simulink model "untitled"  (Simulink 8.7)
settings: Solver=VariableStepAuto  StartTime=0.0  StopTime=3  RelTol=1e-3
libraries: simulink x8
settings Model: Creator=33105  LastModifiedBy=33105
settings DataIOCC: LimitDataPoints=off  SaveFormat=Dataset
settings DebuggingCC: UnderspecifiedInitializationDetection=Simplified  MergeDetectMultiDrivingBlocksExec=error
settings HardwareCC: ProdBitPerPointer=64  ProdLargestAtomicFloat=Float  ProdIntDivRoundTo=Zero  ProdEndianess=LittleEndian  ProdWordSize=64  ProdHWDeviceType=Intel->x86-64 (Windows64)
settings ModelReferenceCC: PropagateSignalLabelsOutOfModel=on
settings ConfigComp: CovModelRefEnable=off

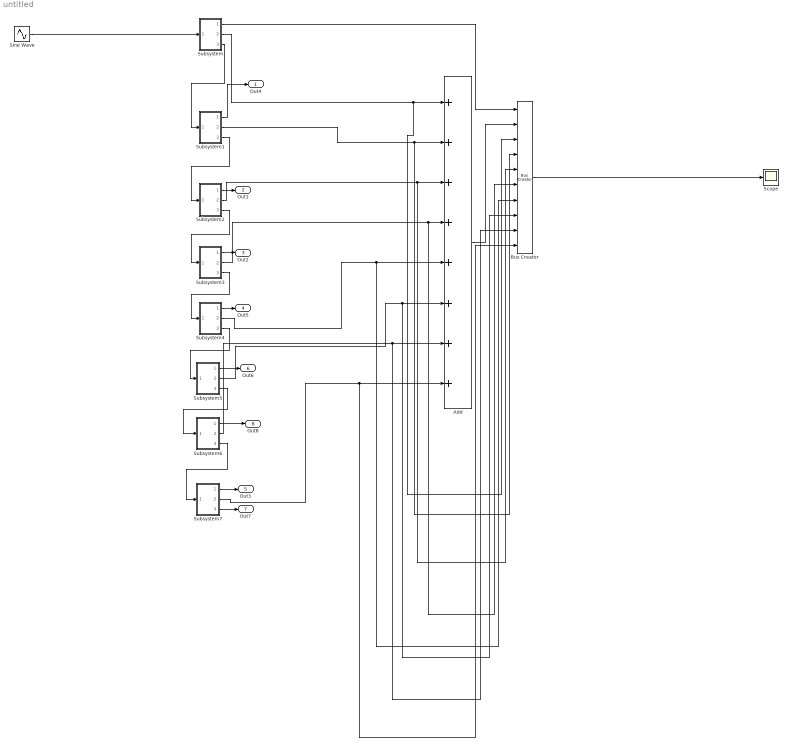
== system untitled ==
  Add : Sum  Inputs=++++++++
  Bus Creator : BusCreator  Inputs=10
  Scope : Scope
  Sine Wave : Sin  Amplitude=8  SampleTime=0
  Subsystem : Subsystem
  Subsystem1 : Subsystem
  Subsystem2 : Subsystem
  Subsystem3 : Subsystem
  Subsystem4 : Subsystem
  Subsystem5 : Subsystem
  Subsystem6 : Subsystem
  Subsystem7 : Subsystem
  Out4 : Outport
  Out1 : Outport  Port=2
  Out2 : Outport  Port=3
  Out5 : Outport  Port=4
  Out3 : Outport  Port=5
  Out6 : Outport  Port=6
  Out7 : Outport  Port=7
  Out8 : Outport  Port=8
  wires:
  Sine Wave/1 -> Subsystem/1(In1)
  Subsystem/2(Out2) -> Bus Creator/3, Add/1
  Subsystem/3(Out3) -> Subsystem1/1(In1)
  Subsystem1/1(Out1) -> Out4/1
  Subsystem1/2(Out2) -> Bus Creator/4, Add/2
  Subsystem1/3(Out3) -> Subsystem2/1(In1)
  Subsystem2/2(Out2) -> Bus Creator/5, Add/3
  Subsystem2/3(Out3) -> Subsystem3/1(In1)
  Subsystem3/2(Out2) -> Bus Creator/6, Add/4
  Subsystem3/3(Out3) -> Subsystem4/1(In1)
  Subsystem4/2(Out2) -> Bus Creator/7, Add/5
  Subsystem2/1(Out1) -> Out1/1
  Subsystem3/1(Out1) -> Out2/1
  Subsystem4/1(Out1) -> Out5/1
  Bus Creator/1 -> Scope/1
  Subsystem/1(Out1) -> Bus Creator/1
  Add/1 -> Bus Creator/2
  Subsystem4/3(Out3) -> Subsystem5/1(In1)
  Subsystem5/2(Out2) -> Bus Creator/8, Add/6
  Subsystem5/3(Out3) -> Subsystem6/1(In1)
  Subsystem5/1(Out1) -> Out6/1
  Subsystem6/2(Out2) -> Bus Creator/9, Add/7
  Subsystem6/3(Out3) -> Subsystem7/1(In1)
  Subsystem6/1(Out1) -> Out8/1
  Subsystem7/1(Out1) -> Out3/1
  Subsystem7/3(Out3) -> Out7/1
  Subsystem7/2(Out2) -> Bus Creator/10, Add/8

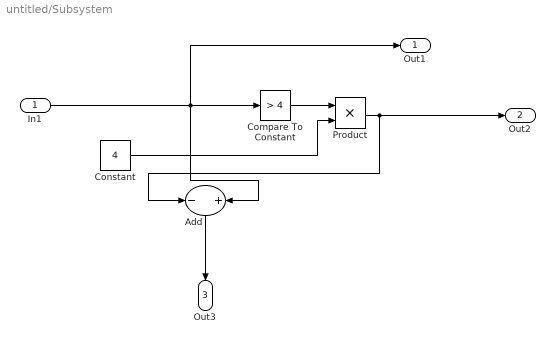
== system untitled/Subsystem ==
  In1 : Inport
  Add : Sum  Inputs=-+
  Compare To Constant : simulink/Logic and Bit Operations/Compare To Constant  relop=>  const=4  OutDataTypeStr=uint8
  Constant : Constant  Value=4
  Product : Product
  Out1 : Outport
  Out2 : Outport  Port=2
  Out3 : Outport  Port=3
  wires:
  Compare To Constant/1 -> Product/1
  Add/1 -> Out3/1
  Product/1 -> Out2/1, Add/1
  In1/1 -> Out1/1, Add/2, Compare To Constant/1
  Constant/1 -> Product/2

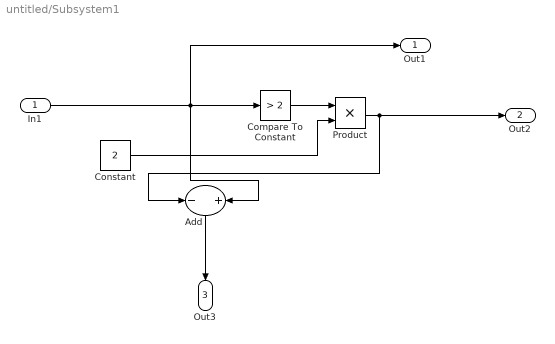
== system untitled/Subsystem1 ==
  In1 : Inport
  Add : Sum  Inputs=-+
  Compare To Constant : simulink/Logic and Bit Operations/Compare To Constant  relop=>  const=2  OutDataTypeStr=uint8
  Constant : Constant  Value=2
  Product : Product
  Out1 : Outport
  Out2 : Outport  Port=2
  Out3 : Outport  Port=3
  wires:
  Compare To Constant/1 -> Product/1
  Add/1 -> Out3/1
  Product/1 -> Out2/1, Add/1
  In1/1 -> Out1/1, Add/2, Compare To Constant/1
  Constant/1 -> Product/2

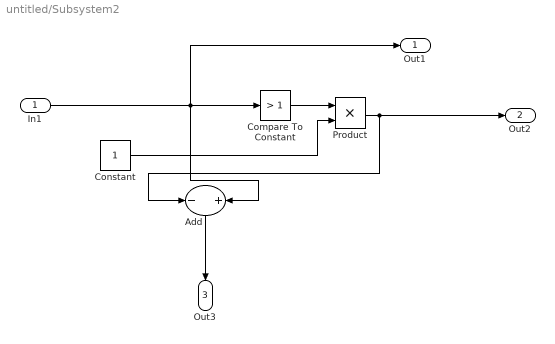
== system untitled/Subsystem2 ==
  In1 : Inport
  Add : Sum  Inputs=-+
  Compare To Constant : simulink/Logic and Bit Operations/Compare To Constant  relop=>  const=1  OutDataTypeStr=uint8
  Constant : Constant
  Product : Product
  Out1 : Outport
  Out2 : Outport  Port=2
  Out3 : Outport  Port=3
  wires:
  Compare To Constant/1 -> Product/1
  Add/1 -> Out3/1
  Product/1 -> Out2/1, Add/1
  In1/1 -> Out1/1, Add/2, Compare To Constant/1
  Constant/1 -> Product/2

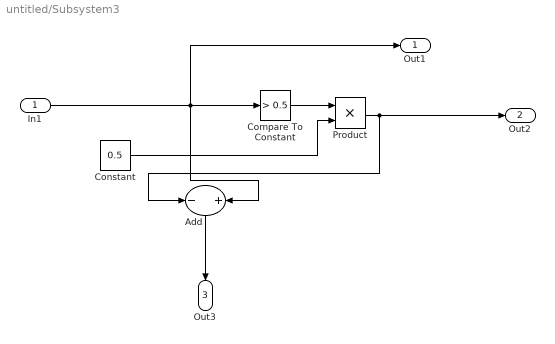
== system untitled/Subsystem3 ==
  In1 : Inport
  Add : Sum  Inputs=-+
  Compare To Constant : simulink/Logic and Bit Operations/Compare To Constant  relop=>  const=0.5  OutDataTypeStr=uint8
  Constant : Constant  Value=0.5
  Product : Product
  Out1 : Outport
  Out2 : Outport  Port=2
  Out3 : Outport  Port=3
  wires:
  Compare To Constant/1 -> Product/1
  Add/1 -> Out3/1
  Product/1 -> Out2/1, Add/1
  In1/1 -> Out1/1, Add/2, Compare To Constant/1
  Constant/1 -> Product/2

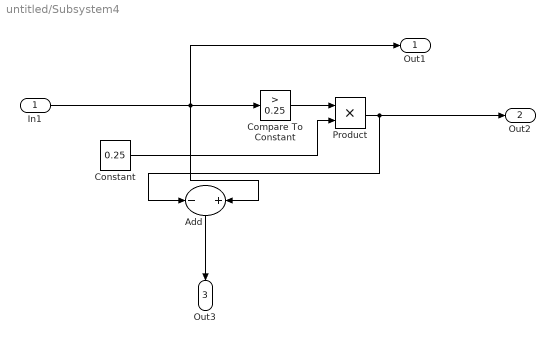
== system untitled/Subsystem4 ==
  In1 : Inport
  Add : Sum  Inputs=-+
  Compare To Constant : simulink/Logic and Bit Operations/Compare To Constant  relop=>  const=0.25  OutDataTypeStr=uint8
  Constant : Constant  Value=0.25
  Product : Product
  Out1 : Outport
  Out2 : Outport  Port=2
  Out3 : Outport  Port=3
  wires:
  Compare To Constant/1 -> Product/1
  Add/1 -> Out3/1
  Product/1 -> Out2/1, Add/1
  In1/1 -> Out1/1, Add/2, Compare To Constant/1
  Constant/1 -> Product/2

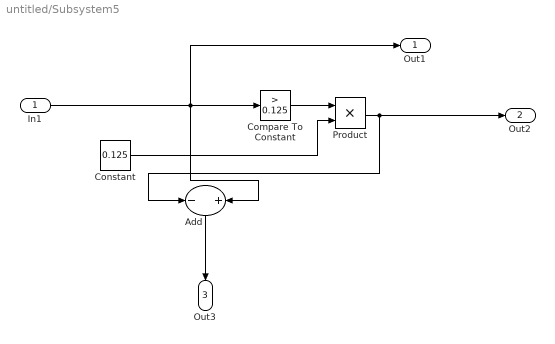
== system untitled/Subsystem5 ==
  In1 : Inport
  Add : Sum  Inputs=-+
  Compare To Constant : simulink/Logic and Bit Operations/Compare To Constant  relop=>  const=0.125  OutDataTypeStr=uint8
  Constant : Constant  Value=0.125
  Product : Product
  Out1 : Outport
  Out2 : Outport  Port=2
  Out3 : Outport  Port=3
  wires:
  Compare To Constant/1 -> Product/1
  Add/1 -> Out3/1
  Product/1 -> Out2/1, Add/1
  In1/1 -> Out1/1, Add/2, Compare To Constant/1
  Constant/1 -> Product/2

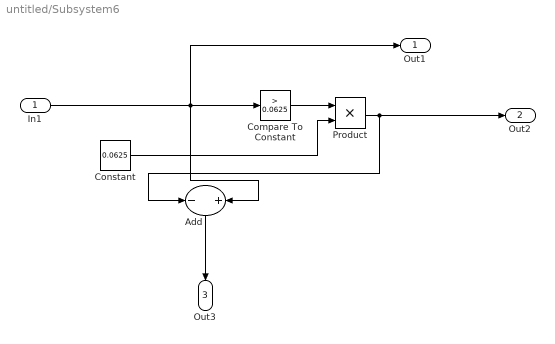
== system untitled/Subsystem6 ==
  In1 : Inport
  Add : Sum  Inputs=-+
  Compare To Constant : simulink/Logic and Bit Operations/Compare To Constant  relop=>  const=0.0625  OutDataTypeStr=uint8
  Constant : Constant  Value=0.0625
  Product : Product
  Out1 : Outport
  Out2 : Outport  Port=2
  Out3 : Outport  Port=3
  wires:
  Compare To Constant/1 -> Product/1
  Add/1 -> Out3/1
  Product/1 -> Out2/1, Add/1
  In1/1 -> Out1/1, Add/2, Compare To Constant/1
  Constant/1 -> Product/2

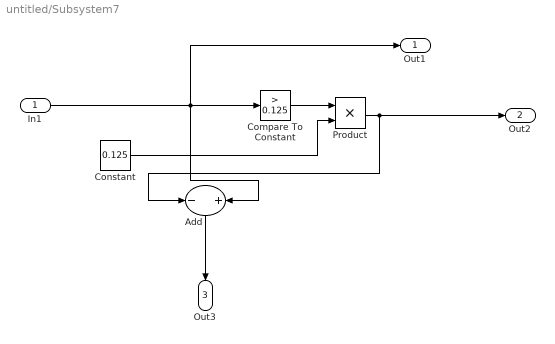
== system untitled/Subsystem7 ==
  In1 : Inport
  Add : Sum  Inputs=-+
  Compare To Constant : simulink/Logic and Bit Operations/Compare To Constant  relop=>  const=0.125  OutDataTypeStr=uint8
  Constant : Constant  Value=0.125
  Product : Product
  Out1 : Outport
  Out2 : Outport  Port=2
  Out3 : Outport  Port=3
  wires:
  Compare To Constant/1 -> Product/1
  Add/1 -> Out3/1
  Product/1 -> Out2/1, Add/1
  In1/1 -> Out1/1, Add/2, Compare To Constant/1
  Constant/1 -> Product/2
